simulink model "Modelo_Fuzzy_Manual"  (R2015b)
settings: Solver=ode1  StartTime=0.0  StopTime=tfin  FixedStep=0.05  RelTol=1e-5  AbsTol=1e-15
undefined symbols (not defined in the file): ACSP, ILSnoise, ParamFuzzy, wind
(part 1 of 2)
settings Model: Creator=cpoh  LastModifiedBy=CPOH

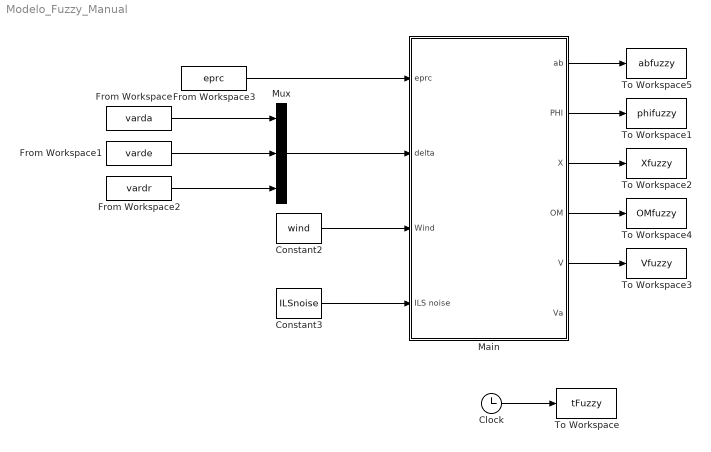
== system Modelo_Fuzzy_Manual ==
  Clock : Clock
  Constant2 : Constant  Value=wind
  Constant3 : Constant  Value=ILSnoise
  From Workspace : FromWorkspace  VariableName=varda  SampleTime=0.05
  From Workspace1 : FromWorkspace  VariableName=varde  SampleTime=0.05
  From Workspace2 : FromWorkspace  VariableName=vardr  SampleTime=0.05
  From Workspace3 : FromWorkspace  VariableName=eprc  SampleTime=0.05
  Main : Subsystem
  Mux : Mux  Inputs=3
  To Workspace : ToWorkspace  VariableName=tFuzzy  SampleTime=-1
  To Workspace1 : ToWorkspace  VariableName=phifuzzy  SampleTime=-1
  To Workspace2 : ToWorkspace  VariableName=Xfuzzy  SampleTime=-1
  To Workspace3 : ToWorkspace  VariableName=Vfuzzy  SampleTime=-1
  To Workspace4 : ToWorkspace  VariableName=OMfuzzy  SampleTime=-1
  To Workspace5 : ToWorkspace  VariableName=abfuzzy  SampleTime=-1
  wires:
  Clock/1 -> To Workspace/1
  Main/2(PHI) -> To Workspace1/1
  Constant3/1 -> Main/4(ILS noise)
  Constant2/1 -> Main/3(Wind)
  Mux/1 -> Main/2(delta)
  From Workspace2/1 -> Mux/3
  From Workspace1/1 -> Mux/2
  From Workspace/1 -> Mux/1
  From Workspace3/1 -> Main/1(eprc)
  Main/3(X) -> To Workspace2/1
  Main/5(V) -> To Workspace3/1
  Main/4(OM) -> To Workspace4/1
  Main/1(ab) -> To Workspace5/1

== system Modelo_Fuzzy_Manual/Main ==
  eprc : Inport
  delta : Inport  Port=2
  Wind : Inport  Port=3
  ILS noise : Inport  Port=4
  A310 Model : Subsystem
  Engines and Actuators : Subsystem
  Gb : Constant  Value=ACSP.U0.wind
  Sum3 : Sum  Inputs=++|
  ab : Outport
  PHI : Outport  Port=2
  X : Outport  Port=3
  OM : Outport  Port=4
  V : Outport  Port=5
  Va : Outport  Port=6
  wires:
  eprc/1 -> Engines and Actuators/1(eprc)
  delta/1 -> Engines and Actuators/2(deflections)
  Engines and Actuators/1(states) -> [xEA]
  Engines and Actuators/2(U) -> A310 Model/1(U)
  Wind/1 -> Sum3/2
  Sum3/1 -> A310 Model/2(Wind)
  Gb/1 -> Sum3/1
  ILS noise/1 -> A310 Model/3(ILSnoise)
  A310 Model/3(PHI) -> PHI/1
  A310 Model/7(Va) -> Va/1
  A310 Model/6(V) -> V/1
  A310 Model/5(OM) -> OM/1
  A310 Model/4(X) -> X/1
  A310 Model/1(ab) -> ab/1

== system Modelo_Fuzzy_Manual/Main/A310 Model ==
  U : Inport
  Wind : Inport  Port=2
  ILSnoise : Inport  Port=3
  Dynamics : Subsystem
  Forces and Momments : Subsystem
  Kinematics : Subsystem
  Mux : Mux  Inputs=2
  Selector10 : Selector  InputPortWidth=3  IndexOptions=Index vector (dialog)  Indices=3  OutputSizes=1
  Trajectory : Subsystem
  WIND : Subsystem
  quat 2 PHI : Subsystem
  ab : Outport
  Nxyz : Outport  Port=2
  PHI : Outport  Port=3
  X : Outport  Port=4
  OM : Outport  Port=5
  V : Outport  Port=6
  Va : Outport  Port=7
  wires:
  Forces and Momments/1(F) -> Dynamics/1(F)
  Forces and Momments/3(M) -> Dynamics/2(M)
  Dynamics/1(V) -> V/1, WIND/1(V), Kinematics/1(V)
  Dynamics/2(OM) -> OM/1, Trajectory/5(OM), Forces and Momments/6(OM), Kinematics/2(OM)
  WIND/1(alpha) -> Mux/1
  WIND/2(beta) -> Mux/2
  Mux/1 -> ab/1, Forces and Momments/1(ab)
  U/1 -> Forces and Momments/2(U)
  WIND/3(Va) -> Va/1, Forces and Momments/3(Va)
  Wind/1 -> WIND/2(WIND)
  WIND/4(qd) -> Forces and Momments/4(qd)
  Kinematics/2(Xdot) -> Trajectory/3(Xdot)
  Kinematics/1(X) -> X/1, Trajectory/2(X)
  Kinematics/3(Quat) -> quat 2 PHI/1(quat)
  ILSnoise/1 -> Trajectory/1(ILSnoise)
  quat 2 PHI/1(PHI) -> PHI/1, Trajectory/4(PHI)
  Forces and Momments/2(Nxyz) -> Nxyz/1
  Selector10/1 -> Forces and Momments/5(HLG)
  Trajectory/2(xyzLG) -> Selector10/1

== system Modelo_Fuzzy_Manual/Main/Engines and Actuators ==
  eprc : Inport
  deflections : Inport  Port=2
  Actuators : Subsystem
  Engines : Subsystem
  Mux : Mux  Inputs=2
  Mux1 : Mux  Inputs=2
  Scope : Scope  NumInputPorts=2
  Sum3 : Sum  Inputs=|++
  delta0 : Constant  Value=ACSP.U0.delta
  epr0 : Constant  Value=ACSP.U0.epr
  states : Outport
  U : Outport  Port=2
  wires:
  Actuators/1(delta) -> Sum3/1, Mux1/2
  Engines/1(TH) -> Mux/1
  eprc/1 -> Engines/2(eprc)
  deflections/1 -> Actuators/1(deltac)
  epr0/1 -> Engines/1(epr0)
  Mux/1 -> U/1
  Engines/2(epr) -> Mux1/1  "EPR"
  Mux1/1 -> states/1
  Sum3/1 -> Scope/1, Mux/2
  delta0/1 -> Sum3/2

== system Modelo_Fuzzy_Manual/Main/A310 Model/Dynamics ==
  note: F =mass*(Vdot + OM x V)
  note: M = I*OMdot + OM x (I*OM)
  F : Inport
  M : Inport  Port=2
  CP1 : Subsystem
      mask Display:
      | fprintf('CROSS \n PRODUCT');
      | color('red');
      | fprintf('\n\n');
      | fprintf(' \n \n \n z=x^y');
      | %text(3,1,'PRODUCT');
      | %text(5,1,'z=x^y');
  CP2 : Subsystem
      mask Display:
      | fprintf('CROSS \n PRODUCT');
      | color('red');
      | fprintf('\n\n');
      | fprintf(' \n \n \n z=x^y');
      | %text(3,1,'PRODUCT');
      | %text(5,1,'z=x^y');
  Inertia : Gain  Gain=ACSP.MIG.I  Multiplication=Matrix(K*u)
  Inertia^-1 : Gain  Gain=ACSP.MIG.J  Multiplication=Matrix(K*u)
  Int_OM : Integrator  InitialCondition=ACSP.X0.OM  ContinuousStateAttributes='OM'
  Int_V : Integrator  InitialCondition=ACSP.X0.V  ContinuousStateAttributes='V'
  Mass^-1 : Gain  Gain=1/ACSP.MIG.mass
  Sum : Sum  Inputs=|+-
  Sum1 : Sum  Inputs=-+|
  V : Outport
  OM : Outport  Port=2
  wires:
  Int_V/1 -> CP2/2(y), V/1
  Sum1/1 -> Int_V/1
  Sum/1 -> Inertia^-1/1
  M/1 -> Sum/1
  Inertia^-1/1 -> Int_OM/1
  F/1 -> Mass^-1/1
  Int_OM/1 -> CP1/1(x), Inertia/1, CP2/1(x), OM/1
  CP2/1(z) -> Sum1/1
  CP1/1(z) -> Sum/2
  Mass^-1/1 -> Sum1/2
  Inertia/1 -> CP1/2(y)

== system Modelo_Fuzzy_Manual/Main/A310 Model/Forces and Momments ==
  ab : Inport
  U : Inport  Port=2
  Va : Inport  Port=3
  qd : Inport  Port=4
  HLG : Inport  Port=5
  OM : Inport  Port=6
  Bus Creator : BusCreator  Inputs=10
  Demux1 : Demux  Outputs=3
  Demux2 : Demux  Outputs=3
  Demux3 : Demux  Outputs=2
  Forces : Subsystem
  Moments : Subsystem
  S : Gain  Gain=ACSP.MIG.Sref
  Selector : Selector  InputPortWidth=4  IndexOptions=Index vector (dialog)  Indices=[2 3 4]  OutputSizes=1
  Selector1 : Selector  InputPortWidth=4  IndexOptions=Index vector (dialog)  Indices=[1]  OutputSizes=1
  F : Outport
  Nxyz : Outport  Port=2
  M : Outport  Port=3
  wires:
  Forces/3(Nxyz) -> Nxyz/1
  Selector1/1 -> Moments/4(TH), Forces/2(TH)
  Forces/2(F) -> F/1
  S/1 -> Moments/3(qS), Forces/3(qS)
  Forces/1(Fa) -> Moments/2(Fa)
  U/1 -> Selector/1, Selector1/1
  Selector/1 -> Demux2/1
  Moments/1(M) -> M/1
  Bus Creator/1 -> Moments/1(E), Forces/1(E)
  Demux1/1 -> Bus Creator/3  "p"
  Demux1/2 -> Bus Creator/4  "q"
  Demux1/3 -> Bus Creator/5  "r"
  Demux3/2 -> Bus Creator/2  "beta"
  Demux2/3 -> Bus Creator/10  "dr"
  Demux2/2 -> Bus Creator/9  "de"
  Demux2/1 -> Bus Creator/8  "da"
  Va/1 -> Bus Creator/6  "Va"
  HLG/1 -> Bus Creator/7  "Hlg"
  OM/1 -> Demux1/1
  qd/1 -> S/1
  Demux3/1 -> Bus Creator/1  "alpha"
  ab/1 -> Demux3/1  "alpha"

== system Modelo_Fuzzy_Manual/Main/A310 Model/Kinematics ==
  V : Inport
  OM : Inport  Port=2
  Gain : Gain  Gain=0.5
  Int_PHI1 : Integrator  InitialCondition=ACSP.X0.QUAT  ContinuousStateAttributes='QUAT'
  Int_X1 : Integrator  InitialCondition=ACSP.X0.X  ContinuousStateAttributes='X'
  R(QUAT) : Subsystem
      mask Display:
      | fprintf('MATRIX \n PRODUCT');
      | color('red');
      | fprintf('\n\n');
      | fprintf(' \n \n \n z=M(x)*y');
  Rotations and transformations matrices in quaternions : Subsystem
  T(QUAT) : Subsystem
      mask Display:
      | fprintf('MATRIX \n PRODUCT');
      | color('red');
      | fprintf('\n\n');
      | fprintf(' \n \n \n z=M(x)*y');
  X : Outport
  Xdot : Outport  Port=2
  Quat : Outport  Port=3
  tag scope: QV2B=global
  wires:
  Int_PHI1/1 -> Quat/1, Rotations and transformations matrices in quaternions/1(QUAT)
  R(QUAT)/1(z) -> Xdot/1, Int_X1/1
  Rotations and transformations matrices in quaternions/3(QB2V) -> R(QUAT)/1(x)
  Rotations and transformations matrices in quaternions/1(TQUAT) -> T(QUAT)/1(x)
  Rotations and transformations matrices in quaternions/2(QV2B) -> [QV2B]
  Gain/1 -> Int_PHI1/1
  T(QUAT)/1(z) -> Gain/1
  OM/1 -> T(QUAT)/2(y)
  V/1 -> R(QUAT)/2(y)
  Int_X1/1 -> X/1

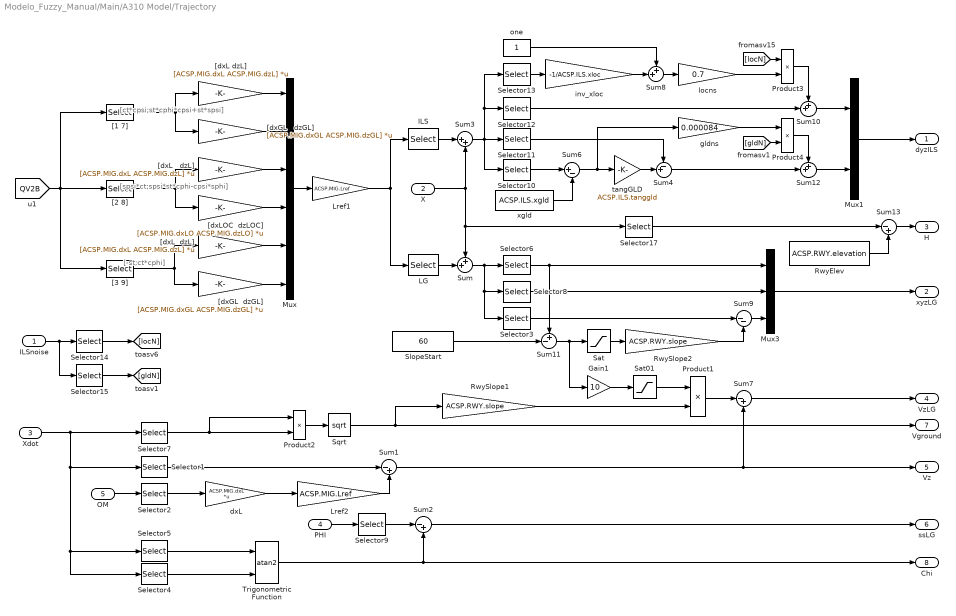
== system Modelo_Fuzzy_Manual/Main/A310 Model/Trajectory ==
  note: [-st;ct*cphi]
  note: [ct*cpsi;st*cphi*cpsi+st*spsi]
  note: [spsi*ct;spsi*st*cphi-cpsi*sphi]
  ILSnoise : Inport
  X : Inport  Port=2
  Xdot : Inport  Port=3
  PHI : Inport  Port=4
  OM : Inport  Port=5
  Gain1 : Gain  Gain=10
  ILS : Selector  InputPortWidth=6  IndexOptions=Index vector (dialog)  Indices=[2 4 6]  OutputSizes=1
  LG : Selector  InputPortWidth=6  IndexOptions=Index vector (dialog)  Indices=[1 3 5]  OutputSizes=1
  Lref1 : Gain  Gain=ACSP.MIG.Lref
  Lref2 : Gain  Gain=ACSP.MIG.Lref
  Mux : Mux  Inputs=6
  Mux1 : Mux  Inputs=2
  Mux3 : Mux  Inputs=3
  Product{1..4} (4 alike) : Product  SaturateOnIntegerOverflow=on  RndMeth=Zero  InputSameDT=on  OutDataTypeStr=Inherit: Same as first input
  RwyElev : Constant  Value=ACSP.RWY.elevation
  RwySlope1 : Gain  Gain=ACSP.RWY.slope
  RwySlope2 : Gain  Gain=ACSP.RWY.slope
  Sat : Saturate  UpperLimit=1000  LowerLimit=0
  Sat01 : Saturate  UpperLimit=1  LowerLimit=0
  Selector{1,3,9,11,17} (5 alike) : Selector  InputPortWidth=3  IndexOptions=Index vector (dialog)  Indices=3  OutputSizes=1
  Selector{4,6..7,10,13} (5 alike) : Selector  InputPortWidth=3  IndexOptions=Index vector (dialog)  Indices=1  OutputSizes=1
  Selector{2,5,8,12} (4 alike) : Selector  InputPortWidth=3  IndexOptions=Index vector (dialog)  Indices=2  OutputSizes=1
  Selector14 : Selector  InputPortWidth=2  IndexOptions=Index vector (dialog)  Indices=1  OutputSizes=1
  Selector15 : Selector  InputPortWidth=2  IndexOptions=Index vector (dialog)  Indices=2  OutputSizes=1
  SlopeStart : Constant  Value=60
  Sqrt : Sqrt  SaturateOnIntegerOverflow=on
  Sum{,8,10,12} (4 alike) : Sum  Inputs=++|
  Sum{1..2,7,13} (4 alike) : Sum  Inputs=|-+
  Sum11 : Sum  Inputs=+-|
  Sum3 : Sum  Inputs=|++
  Sum4 : Sum  Inputs=-+|
  Sum6 : Sum  Inputs=|+-
  Sum9 : Sum  Inputs=|--
  Trigonometric Function : Trigonometry  Operator=atan2
  "[1 7]" : Selector  InputPortWidth=9  IndexOptions=Index vector (dialog)  Indices=[1 7]  OutputSizes=1
  "[2 8]" : Selector  InputPortWidth=9  IndexOptions=Index vector (dialog)  Indices=[2 8]  OutputSizes=1
  "[3 9]" : Selector  InputPortWidth=9  IndexOptions=Index vector (dialog)  Indices=[3 9]  OutputSizes=1
  "[dxGL   dzGL]" : Gain  Gain=[ACSP.MIG.dxGL ACSP.MIG.dzGL]  Multiplication=Matrix(K*u)
  "[dxGL  dzGL]" : Gain  Gain=[ACSP.MIG.dxGL ACSP.MIG.dzGL]  Multiplication=Matrix(K*u)
  "[dxL   dzL]" : Gain  Gain=[ACSP.MIG.dxL ACSP.MIG.dzL]  Multiplication=Matrix(K*u)
  "[dxL  dzL]" : Gain  Gain=[ACSP.MIG.dxL ACSP.MIG.dzL]  Multiplication=Matrix(K*u)
  "[dxL dzL]" : Gain  Gain=[ACSP.MIG.dxL ACSP.MIG.dzL]  Multiplication=Matrix(K*u)
  "[dxLOC  dzLOC]" : Gain  Gain=[ACSP.MIG.dxLO ACSP.MIG.dzLO]  Multiplication=Matrix(K*u)
  dxL : Gain  Gain=ACSP.MIG.dxL  Multiplication=Matrix(K*u)
  gldns : Gain  Gain=0.000084
  inv_xloc : Gain  Gain=-1/ACSP.ILS.xloc
  locns : Gain  Gain=0.7
  one : Constant
  tangGLD : Gain  Gain=ACSP.ILS.tanggld
  xgld : Constant  Value=ACSP.ILS.xgld
  dyzILS : Outport
  xyzLG : Outport  Port=2
  H : Outport  Port=3
  VzLG : Outport  Port=4
  Vz : Outport  Port=5
  ssLG : Outport  Port=6
  Vground : Outport  Port=7
  Chi : Outport  Port=8
  wires:
  Xdot/1 -> Selector1/1, Selector4/1, Selector5/1, Selector7/1
  OM/1 -> Selector2/1
  Selector2/1 -> dxL/1
  dxL/1 -> Lref2/1
  Lref2/1 -> Sum1/2
  Sum1/1 -> Vz/1, Sum7/2
  [QV2B] -> "[1 7]"/1, "[3 9]"/1, "[2 8]"/1
  Selector1/1 -> Sum1/1
  Selector5/1 -> Trigonometric Function/1
  Trigonometric Function/1 -> Sum2/2, Chi/1
  "[1 7]"/1 -> "[dxL dzL]"/1, "[dxGL   dzGL]"/1
  Product2/1 -> Sqrt/1
  Selector4/1 -> Trigonometric Function/2
  Selector7/1 -> Product2/2, Product2/1
  Sqrt/1 -> Vground/1, RwySlope1/1
  "[2 8]"/1 -> "[dxL   dzL]"/1, "[dxLOC  dzLOC]"/1
  PHI/1 -> Selector9/1
  Selector9/1 -> Sum2/1
  Sum2/1 -> ssLG/1
  "[3 9]"/1 -> "[dxL  dzL]"/1, "[dxGL  dzGL]"/1
  "[dxL dzL]"/1 -> Mux/1
  "[dxGL   dzGL]"/1 -> Mux/2
  "[dxL   dzL]"/1 -> Mux/3
  "[dxLOC  dzLOC]"/1 -> Mux/4
  "[dxL  dzL]"/1 -> Mux/5
  "[dxGL  dzGL]"/1 -> Mux/6
  Mux/1 -> Lref1/1
  Lref1/1 -> LG/1, ILS/1
  ILS/1 -> Sum3/1
  Sum3/1 -> Selector10/1, Selector11/1, Selector12/1, Selector13/1
  Sum6/1 -> gldns/1, tangGLD/1
  Selector10/1 -> Sum6/1
  xgld/1 -> Sum6/2
  Mux1/1 -> dyzILS/1
  Selector12/1 -> Sum10/2
  Selector11/1 -> Sum4/1
  tangGLD/1 -> Sum4/2
  Sum4/1 -> Sum12/2
  LG/1 -> Sum/2
  X/1 -> Selector17/1, Sum/1, Sum3/2
  Sum/1 -> Selector6/1, Selector3/1, Selector8/1
  Sat01/1 -> Product1/1
  RwySlope1/1 -> Product1/2
  Sum11/1 -> Gain1/1, Sat/1
  Product1/1 -> Sum7/1
  Sat/1 -> RwySlope2/1
  Mux3/1 -> xyzLG/1
  Selector8/1 -> Mux3/2
  Selector6/1 -> Sum11/1, Mux3/1
  SlopeStart/1 -> Sum11/2
  Sum7/1 -> VzLG/1
  Gain1/1 -> Sat01/1
  Selector13/1 -> inv_xloc/1
  inv_xloc/1 -> Sum8/2
  one/1 -> Sum8/1
  Sum8/1 -> locns/1
  Sum10/1 -> Mux1/1
  locns/1 -> Product3/2
  Product3/1 -> Sum10/1
  Sum12/1 -> Mux1/2
  Product4/1 -> Sum12/1
  gldns/1 -> Product4/1
  ILSnoise/1 -> Selector15/1, Selector14/1
  Selector14/1 -> [locN]
  Selector15/1 -> [gldN]
  [locN] -> Product3/1
  [gldN] -> Product4/2
  RwyElev/1 -> Sum13/2
  Sum13/1 -> H/1
  Selector17/1 -> Sum13/1
  Sum9/1 -> Mux3/3
  RwySlope2/1 -> Sum9/2
  Selector3/1 -> Sum9/1

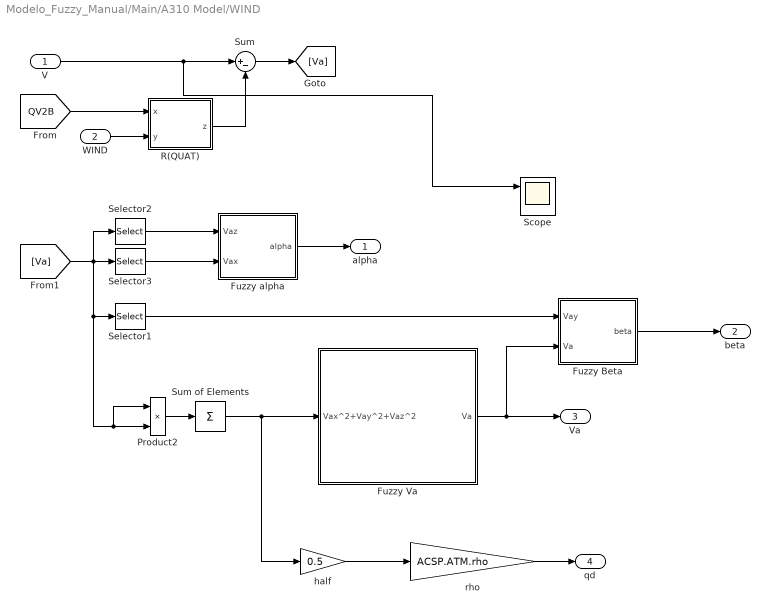
== system Modelo_Fuzzy_Manual/Main/A310 Model/WIND ==
  V : Inport
  WIND : Inport  Port=2
  Fuzzy Beta : Subsystem
  Fuzzy Va : Subsystem
  Fuzzy alpha : Subsystem
  Product2 : Product  SaturateOnIntegerOverflow=on  RndMeth=Zero  InputSameDT=on  OutDataTypeStr=Inherit: Same as first input
  R(QUAT) : Subsystem
      mask Display:
      | fprintf('MATRIX \n PRODUCT');
      | color('red');
      | fprintf('\n\n');
      | fprintf(' \n \n \n z=M(x)*y');
  Scope : Scope  NumInputPorts=2
  Selector1 : Selector  InputPortWidth=3  IndexOptions=Index vector (dialog)  Indices=2  OutputSizes=1
  Selector2 : Selector  InputPortWidth=3  IndexOptions=Index vector (dialog)  Indices=3  OutputSizes=1
  Selector3 : Selector  InputPortWidth=3  IndexOptions=Index vector (dialog)  Indices=1  OutputSizes=1
  Sum : Sum  Inputs=|+-
  Sum of Elements : Sum  Inputs=+
  half : Gain  Gain=0.5  SaturateOnIntegerOverflow=on  OutDataTypeStr=Inherit: Same as input  ParamDataTypeStr=Inherit: Same as input
  rho : Gain  Gain=ACSP.ATM.rho
  alpha : Outport
  beta : Outport  Port=2
  Va : Outport  Port=3
  qd : Outport  Port=4
  wires:
  [QV2B] -> R(QUAT)/1(x)
  WIND/1 -> R(QUAT)/2(y)
  V/1 -> Scope/1, Sum/1
  R(QUAT)/1(z) -> Sum/2
  Sum/1 -> [Va]
  [Va] -> Product2/1, Product2/2, Selector1/1, Selector3/1, Selector2/1
  Product2/1 -> Sum of Elements/1
  Sum of Elements/1 -> half/1, Fuzzy Va/1(Vax^2+Vay^2+Vaz^2)
  Fuzzy Va/1(Va) -> Fuzzy Beta/2(Va), Va/1
  rho/1 -> qd/1
  half/1 -> rho/1
  Selector1/1 -> Fuzzy Beta/1(Vay)
  Fuzzy Beta/1(beta) -> beta/1
  Selector2/1 -> Fuzzy alpha/1(Vaz)
  Selector3/1 -> Fuzzy alpha/2(Vax)
  Fuzzy alpha/1(alpha) -> alpha/1

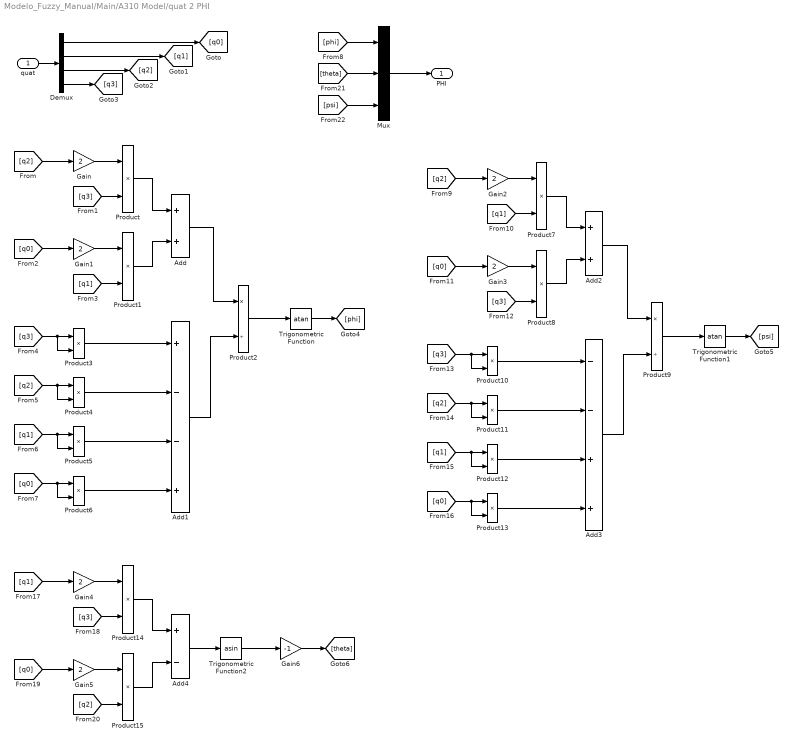
== system Modelo_Fuzzy_Manual/Main/A310 Model/quat 2 PHI ==
  quat : Inport
  Add : Sum
  Add1 : Sum  Inputs=+--+
  Add2 : Sum
  Add3 : Sum  Inputs=--++
  Add4 : Sum  Inputs=+-
  Demux : Demux
  Gain{,1..5} (6 alike) : Gain  Gain=2
  Gain6 : Gain  Gain=-1
  Mux : Mux  Inputs=3
  Product{,1,3..8,10..15} (14 alike) : Product
  Product2 : Product  Inputs=*/
  Product9 : Product  Inputs=*/
  Trigonometric Function : Trigonometry  Operator=atan
  Trigonometric Function1 : Trigonometry  Operator=atan
  Trigonometric Function2 : Trigonometry  Operator=asin
  PHI : Outport
  wires:
  quat/1 -> Demux/1
  Demux/1 -> [q0]
  Demux/2 -> [q1]
  Demux/3 -> [q2]
  Demux/4 -> [q3]
  [q3] -> Product/2
  Gain/1 -> Product/1
  [q2] -> Gain/1
  [q1] -> Product1/2
  Gain1/1 -> Product1/1
  [q0] -> Gain1/1
  Product/1 -> Add/1
  Product1/1 -> Add/2
  [q3] -> Product3/2, Product3/1
  [q2] -> Product4/2, Product4/1
  [q1] -> Product5/2, Product5/1
  [q0] -> Product6/2, Product6/1
  Product3/1 -> Add1/1
  Product4/1 -> Add1/2
  Product5/1 -> Add1/3
  Product6/1 -> Add1/4
  Add1/1 -> Product2/2
  Add/1 -> Product2/1
  Product2/1 -> Trigonometric Function/1
  Trigonometric Function/1 -> [phi]
  Mux/1 -> PHI/1
  [phi] -> Mux/1
  [q1] -> Product7/2
  Gain2/1 -> Product7/1
  [q2] -> Gain2/1
  [q3] -> Product8/2
  Gain3/1 -> Product8/1
  [q0] -> Gain3/1
  Product7/1 -> Add2/1
  Product8/1 -> Add2/2
  [q3] -> Product10/2, Product10/1
  [q2] -> Product11/2, Product11/1
  [q1] -> Product12/2, Product12/1
  [q0] -> Product13/2, Product13/1
  Product10/1 -> Add3/1
  Product11/1 -> Add3/2
  Product12/1 -> Add3/3
  Product13/1 -> Add3/4
  Add3/1 -> Product9/2
  Add2/1 -> Product9/1
  Product9/1 -> Trigonometric Function1/1
  Trigonometric Function1/1 -> [psi]
  [q3] -> Product14/2
  Gain4/1 -> Product14/1
  [q1] -> Gain4/1
  [q2] -> Product15/2
  Gain5/1 -> Product15/1
  [q0] -> Gain5/1
  Product14/1 -> Add4/1
  Product15/1 -> Add4/2
  Add4/1 -> Trigonometric Function2/1
  Trigonometric Function2/1 -> Gain6/1
  Gain6/1 -> [theta]
  [theta] -> Mux/2
  [psi] -> Mux/3

== system Modelo_Fuzzy_Manual/Main/Engines and Actuators/Actuators ==
  deltac : Inport
  Gain2 : Gain  Gain=1./ACSP.ACT.tau
  Int_ASD : Integrator  ContinuousStateAttributes='xASD'
  ML [55 25 30] : Saturate  UpperLimit=ACSP.ACT.ML  LowerLimit=-ACSP.ACT.ML
  RL [60 20 30] : Saturate  UpperLimit=ACSP.ACT.RL  LowerLimit=-ACSP.ACT.RL
  Sum : Sum  Inputs=|+-
  delta : Outport
  wires:
  ML [55 25 30]/1 -> delta/1
  Sum/1 -> Gain2/1
  deltac/1 -> Sum/1
  Int_ASD/1 -> ML [55 25 30]/1, Sum/2
  RL [60 20 30]/1 -> Int_ASD/1
  Gain2/1 -> RL [60 20 30]/1

== system Modelo_Fuzzy_Manual/Main/Engines and Actuators/Engines ==
  epr0 : Inport
  eprc : Inport  Port=2
  EML : Saturate  UpperLimit=ACSP.ENG.UML  LowerLimit=ACSP.ENG.LML
  ERL : Saturate  UpperLimit=ACSP.ENG.RL  LowerLimit=-ACSP.ENG.RL
  Gain1 : Gain  Gain=1/ACSP.ENG.tau
  Gain2 : Gain  Gain=ACSP.ENG.Ga
  Gb : Constant  Value=ACSP.ENG.Gb
  Int_ENG : Integrator  ContinuousStateAttributes='xENG'
  Sum : Sum  Inputs=|+-
  Sum1 : Sum  Inputs=+-|
  Sum2 : Sum  Inputs=|++
  Sum3 : Sum  Inputs=++|
  TH : Outport
  epr : Outport  Port=2
  wires:
  Sum2/1 -> EML/1
  Gb/1 -> Sum3/1
  Gain2/1 -> Sum3/2
  Sum3/1 -> TH/1
  eprc/1 -> Sum/1
  Int_ENG/1 -> Sum2/1, Sum/2
  ERL/1 -> Int_ENG/1
  Gain1/1 -> ERL/1
  Sum/1 -> Gain1/1
  EML/1 -> Sum1/1, Gain2/1
  epr0/1 -> Sum1/2, Sum2/2
  Sum1/1 -> epr/1

== system Modelo_Fuzzy_Manual/Main/A310 Model/Dynamics/CP1 ==
  x : Inport
  y : Inport  Port=2
  Mux : Mux  Inputs=2
  Mux1 : Mux  Inputs=3
  Y1 : Fcn  Expr=u(2)*u(6)-u(3)*u(5)
  Y2 : Fcn  Expr=u(3)*u(4)-u(1)*u(6)
  Y3 : Fcn  Expr=u(1)*u(5)-u(2)*u(4)
  z : Outport
  wires:
  Mux1/1 -> z/1
  Y2/1 -> Mux1/2
  Y1/1 -> Mux1/1
  Y3/1 -> Mux1/3
  y/1 -> Mux/2
  Mux/1 -> Y2/1, Y3/1, Y1/1
  x/1 -> Mux/1

== system Modelo_Fuzzy_Manual/Main/A310 Model/Dynamics/CP2 ==
  x : Inport
  y : Inport  Port=2
  Mux : Mux  Inputs=2
  Mux1 : Mux  Inputs=3
  Y1 : Fcn  Expr=u(2)*u(6)-u(3)*u(5)
  Y2 : Fcn  Expr=u(3)*u(4)-u(1)*u(6)
  Y3 : Fcn  Expr=u(1)*u(5)-u(2)*u(4)
  z : Outport
  wires:
  Mux1/1 -> z/1
  Y2/1 -> Mux1/2
  Y1/1 -> Mux1/1
  Y3/1 -> Mux1/3
  y/1 -> Mux/2
  Mux/1 -> Y2/1, Y3/1, Y1/1
  x/1 -> Mux/1

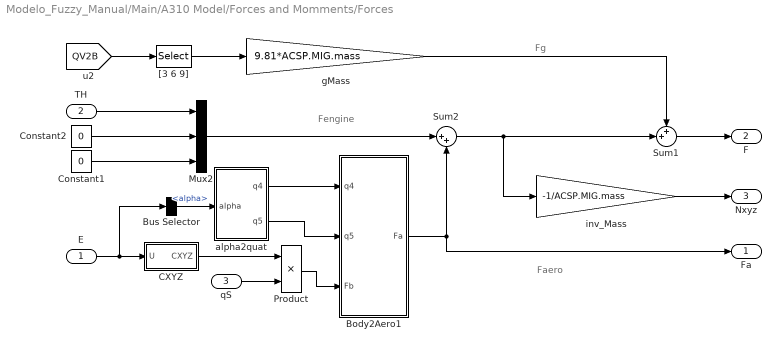
== system Modelo_Fuzzy_Manual/Main/A310 Model/Forces and Momments/Forces ==
  note: Fg
  note: Fengine
  note: Faero
  E : Inport
  TH : Inport  Port=2
  qS : Inport  Port=3
  Body2Aero1 : Subsystem
  Bus Selector : BusSelector  OutputSignals=alpha
  CXYZ : Subsystem
  Constant1 : Constant  Value=0
  Constant2 : Constant  Value=0
  Mux2 : Mux  Inputs=3
  Product : Product  RndMeth=Zero
  Sum1 : Sum  Inputs=++|
  Sum2 : Sum  Inputs=|++
  "[3 6 9]" : Selector  InputPortWidth=9  IndexOptions=Index vector (dialog)  Indices=[3 6 9]  OutputSizes=1
  alpha2quat : Subsystem
  gMass : Gain  Gain=9.81*ACSP.MIG.mass
  inv_Mass : Gain  Gain=-1/ACSP.MIG.mass
  Fa : Outport
  F : Outport  Port=2
  Nxyz : Outport  Port=3
  wires:
  inv_Mass/1 -> Nxyz/1
  Sum2/1 -> Sum1/2, inv_Mass/1
  Mux2/1 -> Sum2/1
  CXYZ/1(CXYZ) -> Product/1
  E/1 -> CXYZ/1(U), Bus Selector/1
  Product/1 -> Body2Aero1/3(Fb)
  qS/1 -> Product/2
  Sum1/1 -> F/1
  "[3 6 9]"/1 -> gMass/1
  [QV2B] -> "[3 6 9]"/1
  Constant1/1 -> Mux2/3
  Constant2/1 -> Mux2/2
  TH/1 -> Mux2/1
  Bus Selector/1 -> alpha2quat/1(alpha)  "<alpha>"
  alpha2quat/1(q4) -> Body2Aero1/1(q4)
  alpha2quat/2(q5) -> Body2Aero1/2(q5)
  gMass/1 -> Sum1/1
  Body2Aero1/1(Fa) -> Fa/1, Sum2/2

== system Modelo_Fuzzy_Manual/Main/A310 Model/Forces and Momments/Moments ==
  note: Ma
  note: Mengine
  note: MFaero
  E : Inport
  Fa : Inport  Port=2
  qS : Inport  Port=3
  TH : Inport  Port=4
  CD0 : Constant  Value=ACSP.MIG.dxG
  CP : Subsystem
      mask Display:
      | fprintf('CROSS \n PRODUCT');
      | color('red');
      | fprintf('\n\n');
      | fprintf(' \n \n \n z=x^y');
      | %text(3,1,'PRODUCT');
      | %text(5,1,'z=x^y');
  Clmn : Subsystem
  Constant{1..4} (4 alike) : Constant  Value=0
  Engine vertical position : Gain  Gain=ACSP.MIG.dzE
  Lref : Gain  Gain=ACSP.MIG.Lref
  Mux1 : Mux  Inputs=3
  Mux2 : Mux  Inputs=3
  Product : Product  RndMeth=Zero
  Sum1 : Sum  Inputs=+++
  M : Outport
  wires:
  E/1 -> Clmn/1(U)
  Clmn/1(Clmn) -> Product/2
  Lref/1 -> M/1
  Mux2/1 -> Sum1/3
  Product/1 -> Sum1/2
  CD0/1 -> Mux1/1
  Constant4/1 -> Mux1/3
  Constant3/1 -> Mux1/2
  CP/1(z) -> Sum1/1
  Mux1/1 -> CP/1(x)
  Fa/1 -> CP/2(y)
  qS/1 -> Product/1
  Constant2/1 -> Mux2/1
  Engine vertical position/1 -> Mux2/2
  TH/1 -> Engine vertical position/1
  Sum1/1 -> Lref/1
  Constant1/1 -> Mux2/3

== system Modelo_Fuzzy_Manual/Main/A310 Model/Kinematics/R(QUAT) ==
  x : Inport
  y : Inport  Port=2
  Mux : Mux  Inputs=2
  Mux1 : Mux  Inputs=3
  Y1 : Fcn  Expr=u(1)*u(10)+u(2)*u(11)+u(3)*u(12)
  Y2 : Fcn  Expr=u(4)*u(10)+u(5)*u(11)+u(6)*u(12)
  Y3 : Fcn  Expr=u(7)*u(10)+u(8)*u(11)+u(9)*u(12)
  z : Outport
  wires:
  Mux1/1 -> z/1
  Y2/1 -> Mux1/2
  Y1/1 -> Mux1/1
  Y3/1 -> Mux1/3
  y/1 -> Mux/2
  Mux/1 -> Y2/1, Y1/1, Y3/1
  x/1 -> Mux/1

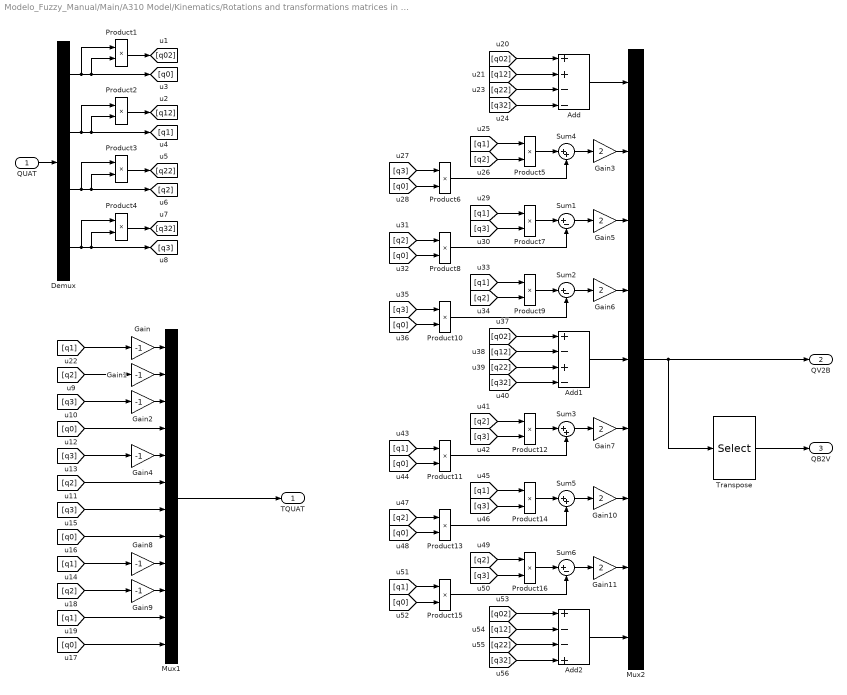
== system Modelo_Fuzzy_Manual/Main/A310 Model/Kinematics/Rotations and transformations matrices in quaternions ==
  QUAT : Inport
  Add : Sum  Inputs=++--
  Add1 : Sum  Inputs=+-+-
  Add2 : Sum  Inputs=+--+
  Demux : Demux
  Gain{,1..2,4,8..9} (6 alike) : Gain  Gain=-1
  Gain{3,5..7,10..11} (6 alike) : Gain  Gain=2
  Mux1 : Mux  Inputs=12
  Mux2 : Mux  Inputs=9
  Product{1..16} (16 alike) : Product  SaturateOnIntegerOverflow=on  RndMeth=Zero  InputSameDT=on  OutDataTypeStr=Inherit: Same as first input
  Sum1 : Sum  Inputs=|+-
  Sum2 : Sum  Inputs=|+-
  Sum3 : Sum  Inputs=|++
  Sum4 : Sum  Inputs=|++
  Sum5 : Sum  Inputs=|++
  Sum6 : Sum  Inputs=|+-
  Transpose : Selector  InputPortWidth=9  IndexOptions=Index vector (dialog)  Indices=[1 4 7 2 5 8 3 6 9]  OutputSizes=1
  TQUAT : Outport
  QV2B : Outport  Port=2
  QB2V : Outport  Port=3
  wires:
  QUAT/1 -> Demux/1
  Demux/1 -> Product1/1, Product1/2, [q0]
  Product1/1 -> [q02]
  Demux/2 -> Product2/1, Product2/2, [q1]
  Product2/1 -> [q12]
  Demux/3 -> Product3/1, Product3/2, [q2]
  Product3/1 -> [q22]
  Demux/4 -> Product4/1, Product4/2, [q3]
  Product4/1 -> [q32]
  Mux1/1 -> TQUAT/1
  Gain/1 -> Mux1/1
  [q1] -> Gain/1
  [q2] -> Gain1/1
  Gain1/1 -> Mux1/2
  [q3] -> Gain2/1
  Gain2/1 -> Mux1/3
  [q3] -> Gain4/1
  [q1] -> Gain8/1
  [q2] -> Gain9/1
  Gain9/1 -> Mux1/10
  [q1] -> Mux1/11
  [q0] -> Mux1/12
  Gain8/1 -> Mux1/9
  [q0] -> Mux1/8
  [q3] -> Mux1/7
  [q2] -> Mux1/6
  Gain4/1 -> Mux1/5
  [q0] -> Mux1/4
  Add/1 -> Mux2/1
  [q32] -> Add/4
  [q22] -> Add/3
  [q12] -> Add/2
  [q02] -> Add/1
  Gain3/1 -> Mux2/2
  Sum4/1 -> Gain3/1
  Product5/1 -> Sum4/1
  [q1] -> Product5/1
  [q2] -> Product5/2
  Product6/1 -> Sum4/2
  [q3] -> Product6/1
  [q0] -> Product6/2
  Gain5/1 -> Mux2/3
  Sum1/1 -> Gain5/1
  Product7/1 -> Sum1/1
  [q1] -> Product7/1
  [q3] -> Product7/2
  Product8/1 -> Sum1/2
  [q2] -> Product8/1
  [q0] -> Product8/2
  Gain6/1 -> Mux2/4
  Sum2/1 -> Gain6/1
  Product9/1 -> Sum2/1
  [q1] -> Product9/1
  [q2] -> Product9/2
  Product10/1 -> Sum2/2
  [q3] -> Product10/1
  [q0] -> Product10/2
  Add1/1 -> Mux2/5
  [q32] -> Add1/4
  [q22] -> Add1/3
  [q12] -> Add1/2
  [q02] -> Add1/1
  Sum3/1 -> Gain7/1
  Product12/1 -> Sum3/1
  [q2] -> Product12/1
  [q3] -> Product12/2
  Product11/1 -> Sum3/2
  [q1] -> Product11/1
  [q0] -> Product11/2
  Gain7/1 -> Mux2/6
  Sum5/1 -> Gain10/1
  Product14/1 -> Sum5/1
  [q1] -> Product14/1
  [q3] -> Product14/2
  Product13/1 -> Sum5/2
  [q2] -> Product13/1
  [q0] -> Product13/2
  Gain10/1 -> Mux2/7
  Sum6/1 -> Gain11/1
  Product16/1 -> Sum6/1
  [q2] -> Product16/1
  [q3] -> Product16/2
  Product15/1 -> Sum6/2
  [q1] -> Product15/1
  [q0] -> Product15/2
  Gain11/1 -> Mux2/8
  Add2/1 -> Mux2/9
  [q32] -> Add2/4
  [q22] -> Add2/3
  [q12] -> Add2/2
  [q02] -> Add2/1
  Mux2/1 -> QV2B/1, Transpose/1
  Transpose/1 -> QB2V/1

== system Modelo_Fuzzy_Manual/Main/A310 Model/Kinematics/T(QUAT) ==
  x : Inport
  y : Inport  Port=2
  Mux : Mux  Inputs=2
  Mux1 : Mux
  Y1 : Fcn  Expr=u(1)*u(13)+u(2)*u(14)+u(3)*u(15)
  Y2 : Fcn  Expr=u(4)*u(13)+u(5)*u(14)+u(6)*u(15)
  Y3 : Fcn  Expr=u(7)*u(13)+u(8)*u(14)+u(9)*u(15)
  Y4 : Fcn  Expr=u(10)*u(13)+u(11)*u(14)+u(12)*u(15)
  z : Outport
  wires:
  Mux1/1 -> z/1
  Y2/1 -> Mux1/2
  Y1/1 -> Mux1/1
  Y3/1 -> Mux1/3
  y/1 -> Mux/2
  Mux/1 -> Y2/1, Y1/1, Y4/1, Y3/1
  x/1 -> Mux/1
  Y4/1 -> Mux1/4

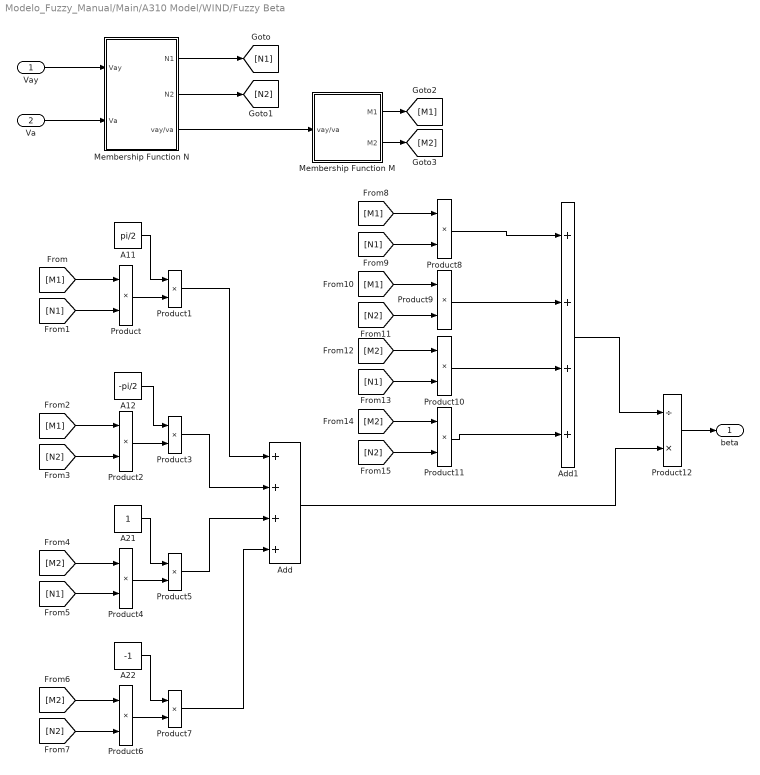
== system Modelo_Fuzzy_Manual/Main/A310 Model/WIND/Fuzzy Beta ==
  Vay : Inport
  Va : Inport  Port=2
  A11 : Constant  Value=pi/2
  A12 : Constant  Value=-pi/2
  A21 : Constant
  A22 : Constant  Value=-1
  Add : Sum  Inputs=++++
  Add1 : Sum  Inputs=++++
  Membership Function M : Subsystem
  Membership Function N : Subsystem
  Product{,1..11} (12 alike) : Product
  Product12 : Product  Inputs=/*
  beta : Outport
  wires:
  Vay/1 -> Membership Function N/1(Vay)
  Va/1 -> Membership Function N/2(Va)
  Membership Function M/2(M2) -> [M2]
  Membership Function M/1(M1) -> [M1]
  Membership Function N/2(N2) -> [N2]
  Membership Function N/1(N1) -> [N1]
  Membership Function N/3(vay/va) -> Membership Function M/1(vay/va)
  A11/1 -> Product1/1
  [M1] -> Product/1
  Product/1 -> Product1/2
  [N1] -> Product/2
  A12/1 -> Product3/1
  [M1] -> Product2/1
  Product2/1 -> Product3/2
  [N2] -> Product2/2
  A21/1 -> Product5/1
  [M2] -> Product4/1
  Product4/1 -> Product5/2
  [N1] -> Product4/2
  A22/1 -> Product7/1
  [M2] -> Product6/1
  Product6/1 -> Product7/2
  [N2] -> Product6/2
  Product1/1 -> Add/1
  Product3/1 -> Add/2
  Product5/1 -> Add/3
  Product7/1 -> Add/4
  [M1] -> Product8/1
  [N1] -> Product8/2
  [M1] -> Product9/1
  [N2] -> Product9/2
  [M2] -> Product11/1
  [N2] -> Product11/2
  Product9/1 -> Add1/2
  Product10/1 -> Add1/3
  Product8/1 -> Add1/1
  Product11/1 -> Add1/4
  Product12/1 -> beta/1
  Add1/1 -> Product12/1
  Add/1 -> Product12/2
  [M2] -> Product10/1
  [N1] -> Product10/2

== system Modelo_Fuzzy_Manual/Main/A310 Model/WIND/Fuzzy Va ==
  Vax^2+Vay^2+Vaz^2 : Inport
  Add : Sum
  Max : Constant  Value=160000
  Membership functions : Subsystem
  Min : Constant  Value=0
  Product : Product
  Product1 : Product
  Va : Outport
  wires:
  Vax^2+Vay^2+Vaz^2/1 -> Membership functions/1(U)
  Max/1 -> Product/1
  Membership functions/1(M1) -> Product/2
  Membership functions/2(M2) -> Product1/1
  Min/1 -> Product1/2
  Product1/1 -> Add/2
  Product/1 -> Add/1
  Add/1 -> Va/1

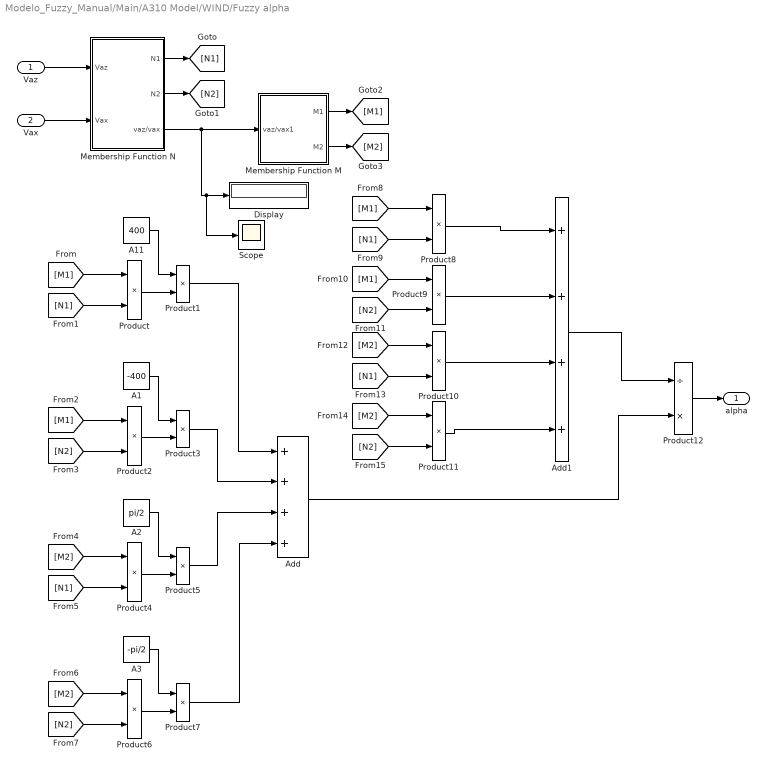
== system Modelo_Fuzzy_Manual/Main/A310 Model/WIND/Fuzzy alpha ==
  Vaz : Inport
  Vax : Inport  Port=2
  A1 : Constant  Value=-400
  A11 : Constant  Value=400
  A2 : Constant  Value=pi/2
  A3 : Constant  Value=-pi/2
  Add : Sum  Inputs=++++
  Add1 : Sum  Inputs=++++
  Display : Display
  Membership Function M : Subsystem
  Membership Function N : Subsystem
  Product{,1..11} (12 alike) : Product
  Product12 : Product  Inputs=/*
  Scope : Scope
  alpha : Outport
  wires:
  Vaz/1 -> Membership Function N/1(Vaz)
  Vax/1 -> Membership Function N/2(Vax)
  Membership Function N/1(N1) -> [N1]
  Membership Function N/2(N2) -> [N2]
  A11/1 -> Product1/1
  [M1] -> Product/1
  Product/1 -> Product1/2
  [N1] -> Product/2
  A1/1 -> Product3/1
  [M1] -> Product2/1
  Product2/1 -> Product3/2
  [N2] -> Product2/2
  A2/1 -> Product5/1
  [M2] -> Product4/1
  Product4/1 -> Product5/2
  [N1] -> Product4/2
  A3/1 -> Product7/1
  [M2] -> Product6/1
  Product6/1 -> Product7/2
  [N2] -> Product6/2
  Product1/1 -> Add/1
  Product3/1 -> Add/2
  Product5/1 -> Add/3
  Product7/1 -> Add/4
  [M1] -> Product8/1
  [N1] -> Product8/2
  [M1] -> Product9/1
  [N2] -> Product9/2
  [M2] -> Product11/1
  Product9/1 -> Add1/2
  Product10/1 -> Add1/3
  Product8/1 -> Add1/1
  Product11/1 -> Add1/4
  Add1/1 -> Product12/1
  Add/1 -> Product12/2
  Product12/1 -> alpha/1
  [N2] -> Product11/2
  [M2] -> Product10/1
  [N1] -> Product10/2
  Membership Function N/3(vaz/vax) -> Scope/1, Display/1, Membership Function M/1(vaz/vax1)
  Membership Function M/1(M1) -> [M1]
  Membership Function M/2(M2) -> [M2]

== system Modelo_Fuzzy_Manual/Main/A310 Model/WIND/R(QUAT) ==
  x : Inport
  y : Inport  Port=2
  Mux : Mux  Inputs=2
  Mux1 : Mux  Inputs=3
  Y1 : Fcn  Expr=u(1)*u(10)+u(2)*u(11)+u(3)*u(12)
  Y2 : Fcn  Expr=u(4)*u(10)+u(5)*u(11)+u(6)*u(12)
  Y3 : Fcn  Expr=u(7)*u(10)+u(8)*u(11)+u(9)*u(12)
  z : Outport
  wires:
  Mux1/1 -> z/1
  Y2/1 -> Mux1/2
  Y1/1 -> Mux1/1
  Y3/1 -> Mux1/3
  y/1 -> Mux/2
  Mux/1 -> Y2/1, Y1/1, Y3/1
  x/1 -> Mux/1

== system Modelo_Fuzzy_Manual/Main/A310 Model/Forces and Momments/Forces/Body2Aero1 ==
  q4 : Inport
  q5 : Inport  Port=2
  Fb : Inport  Port=3
  Mux : Mux  Inputs=[1 1 3]
  Mux3 : Mux  Inputs=3
  Segunda fila : Fcn  Expr=(u(1)^2+u(2)^2)*u(4)
  Tercera fila : Fcn  Expr=-2*u(1)*u(2)*u(3)+(u(1)^2-u(2)^2)*u(5)
  primera fila : Fcn  Expr=(u(1)^2-u(2)^2)*u(3)+2*u(1)*u(2)*u(5)
  Fa : Outport
  wires:
  Fb/1 -> Mux/3
  q4/1 -> Mux/1
  q5/1 -> Mux/2
  Mux/1 -> Tercera fila/1, Segunda fila/1, primera fila/1
  Tercera fila/1 -> Mux3/3
  Segunda fila/1 -> Mux3/2
  primera fila/1 -> Mux3/1
  Mux3/1 -> Fa/1

== system Modelo_Fuzzy_Manual/Main/A310 Model/Forces and Momments/Forces/CXYZ ==
  U : Inport
  Bus Selector : BusSelector  OutputSignals=alpha
  Bus Selector1 : BusSelector  OutputSignals=beta,dr
  Bus Selector2 : BusSelector  OutputSignals=alpha,q,Va,de
  Bus Selector3 : BusSelector  OutputSignals=Hlg
  CL0 : Constant  Value=ACSP.COEF.CL.CL0
  CLa : Gain  Gain=ACSP.COEF.CL.CLa
  CLa3 : Gain  Gain=ACSP.COEF.CL.CLde
  CY_beta : Gain  Gain=ACSP.COEF.CY.CYb
  CY_dr : Gain  Gain=ACSP.COEF.CY.CYdr
  Fuzzy CD (manual) : Subsystem
  Fuzzy CL1 (manual) : Subsystem
  Fuzzy CL2 (manual) : Subsystem
  Gain : Gain  Gain=-1
  Gain1 : Gain  Gain=-1
  Mux : Mux  Inputs=3
  Sum1 : Sum
  Sum3 : Sum  Inputs=++++
  Sum4 : Sum  Inputs=|++
  CXYZ : Outport
  wires:
  Sum4/1 -> Gain1/1
  Sum3/1 -> Sum4/1
  CLa3/1 -> Sum3/4
  Bus Selector2/4 -> CLa3/1  "<de>"
  Mux/1 -> CXYZ/1
  Sum1/1 -> Mux/2
  Gain/1 -> Mux/1
  Gain1/1 -> Mux/3
  CL0/1 -> Sum3/1
  Bus Selector2/1 -> CLa/1  "<alpha>"
  CLa/1 -> Sum3/2
  CY_dr/1 -> Sum1/2
  CY_beta/1 -> Sum1/1
  Bus Selector1/2 -> CY_dr/1  "<dr>"
  Bus Selector1/1 -> CY_beta/1  "<beta>"
  U/1 -> Bus Selector/1, Bus Selector1/1, Bus Selector2/1, Bus Selector3/1
  Bus Selector2/2 -> Fuzzy CL1 (manual)/1(q)  "<q>"
  Bus Selector2/3 -> Fuzzy CL1 (manual)/2(Va)  "<Va>"
  Fuzzy CL1 (manual)/1(CL1) -> Sum3/3
  Bus Selector3/1 -> Fuzzy CL2 (manual)/1(Hlg)  "<Hlg>"
  Fuzzy CL2 (manual)/1(CL2) -> Sum4/2
  Bus Selector/1 -> Fuzzy CD (manual)/1(alpha)  "<alpha>"
  Fuzzy CD (manual)/1(CD) -> Gain/1

== system Modelo_Fuzzy_Manual/Main/A310 Model/Forces and Momments/Forces/alpha2quat ==
  alpha : Inport
  Constant : Constant  Value=-2
  Divide : Product  Inputs=*/
  Trigonometric Function : Trigonometry  Operator=cos
  Trigonometric Function1 : Trigonometry
  q4 : Outport
  q5 : Outport  Port=2
  wires:
  alpha/1 -> Divide/1
  Constant/1 -> Divide/2
  Divide/1 -> Trigonometric Function1/1, Trigonometric Function/1
  Trigonometric Function/1 -> q4/1
  Trigonometric Function1/1 -> q5/1

== system Modelo_Fuzzy_Manual/Main/A310 Model/Forces and Momments/Moments/CP ==
  x : Inport
  y : Inport  Port=2
  Mux : Mux  Inputs=2
  Mux1 : Mux  Inputs=3
  Y1 : Fcn  Expr=u(2)*u(6)-u(3)*u(5)
  Y2 : Fcn  Expr=u(3)*u(4)-u(1)*u(6)
  Y3 : Fcn  Expr=u(1)*u(5)-u(2)*u(4)
  z : Outport
  wires:
  Mux1/1 -> z/1
  Y2/1 -> Mux1/2
  Y1/1 -> Mux1/1
  Y3/1 -> Mux1/3
  y/1 -> Mux/2
  Mux/1 -> Y2/1, Y3/1, Y1/1
  x/1 -> Mux/1

== system Modelo_Fuzzy_Manual/Main/A310 Model/Forces and Momments/Moments/Clmn ==
  U : Inport
  Cl : Subsystem
  Cm : Subsystem
  Cn : Subsystem
  Mux : Mux  Inputs=3
  Clmn : Outport
  wires:
  Mux/1 -> Clmn/1
  Cn/1(Cn) -> Mux/3
  Cm/1(Cm) -> Mux/2
  Cl/1(Cl) -> Mux/1
  U/1 -> Cm/1(U), Cl/1(U), Cn/1(U)

== system Modelo_Fuzzy_Manual/Main/A310 Model/WIND/Fuzzy Beta/Membership Function M ==
  vay/va : Inport
  Add : Sum
  Add1 : Sum
  Constant : Constant
  If : If  IfExpression=u1==0
  If Action Subsystem : Subsystem  TreatAsAtomicUnit=on
  If Action Subsystem1 : Subsystem  TreatAsAtomicUnit=on
  M1 : Outport
  M2 : Outport  Port=2
  wires:
  vay/va/1 -> If Action Subsystem/1(vay/va), If/1
  If/1 -> If Action Subsystem1/Action
  If/2 -> If Action Subsystem/Action
  Constant/1 -> If Action Subsystem1/1(In1)
  If Action Subsystem1/1(M1) -> Add/1
  If Action Subsystem/1(M1) -> Add/2
  If Action Subsystem/2(M2) -> Add1/2
  If Action Subsystem1/2(M2) -> Add1/1
  Add/1 -> M1/1
  Add1/1 -> M2/1

== system Modelo_Fuzzy_Manual/Main/A310 Model/WIND/Fuzzy Beta/Membership Function N ==
  Vay : Inport
  Va : Inport  Port=2
  Add : Sum
  Add1 : Sum  Inputs=-+
  Constant : Constant
  Constant1 : Constant  Value=2
  Constant2 : Constant
  Divide : Product  Inputs=*/
  Divide1 : Product  Inputs=*/
  N1 : Outport
  N2 : Outport  Port=2
  vay/va : Outport  Port=3
  wires:
  Va/1 -> Divide/2
  Vay/1 -> Divide/1
  Divide/1 -> vay/va/1, Add/2
  Constant/1 -> Add/1
  Add/1 -> Divide1/1
  Constant1/1 -> Divide1/2
  Divide1/1 -> Add1/1, N1/1
  Add1/1 -> N2/1
  Constant2/1 -> Add1/2

== system Modelo_Fuzzy_Manual/Main/A310 Model/WIND/Fuzzy Va/Membership functions ==
  U : Inport
  Add : Sum  Inputs=-+
  Constant : Constant  Value=160000
  Constant1 : Constant
  Product : Product  Inputs=*/
  Sqrt : Sqrt  SaturateOnIntegerOverflow=on
  M1 : Outport
  M2 : Outport  Port=2
  wires:
  U/1 -> Sqrt/1
  Sqrt/1 -> Product/1
  Constant/1 -> Product/2
  Product/1 -> Add/1, M1/1
  Constant1/1 -> Add/2
  Add/1 -> M2/1

== system Modelo_Fuzzy_Manual/Main/A310 Model/WIND/Fuzzy alpha/Membership Function M ==
  vaz/vax1 : Inport
  Add3 : Sum
  Add4 : Sum
  Constant3 : Constant
  If : If  IfExpression=u1==0
  If Action Subsystem : Subsystem  TreatAsAtomicUnit=on
  If Action Subsystem1 : Subsystem  TreatAsAtomicUnit=on
  M1 : Outport
  M2 : Outport  Port=2
  wires:
  If/1 -> If Action Subsystem1/Action
  If/2 -> If Action Subsystem/Action
  Constant3/1 -> If Action Subsystem1/1(In1)
  If Action Subsystem1/1(M1) -> Add3/1
  If Action Subsystem1/2(M2) -> Add4/1
  Add3/1 -> M1/1
  Add4/1 -> M2/1
  If Action Subsystem/2(M2) -> Add4/2
  If Action Subsystem/1(M1) -> Add3/2
  vaz/vax1/1 -> If Action Subsystem/1(vaz/vax), If/1

== system Modelo_Fuzzy_Manual/Main/A310 Model/WIND/Fuzzy alpha/Membership Function N ==
  Vaz : Inport
  Vax : Inport  Port=2
  Add : Sum
  Add1 : Sum  Inputs=-+
  Constant : Constant  Value=400
  Constant1 : Constant  Value=800
  Constant2 : Constant
  Divide : Product  Inputs=*/
  Divide1 : Product  Inputs=*/
  N1 : Outport
  N2 : Outport  Port=2
  vaz/vax : Outport  Port=3
  wires:
  Vax/1 -> Divide/2
  Vaz/1 -> Divide/1
  Divide/1 -> vaz/vax/1, Add/2
  Constant/1 -> Add/1
  Add/1 -> Divide1/1
  Constant1/1 -> Divide1/2
  Divide1/1 -> Add1/1, N1/1
  Add1/1 -> N2/1
  Constant2/1 -> Add1/2

== system Modelo_Fuzzy_Manual/Main/A310 Model/Forces and Momments/Forces/CXYZ/Fuzzy CD (manual) ==
  alpha : Inport
  Add : Sum
  Add1 : Sum
  CD0 : Constant  Value=ACSP.COEF.CD.CD0
  CD_alpha : Gain  Gain=ACSP.COEF.CD.CDa
  CD_alpha1 : Gain  Gain=ParamFuzzy.CD.max
  CD_alpha2 : Gain  Gain=ACSP.COEF.CD.CDa2
  CD_alpha3 : Gain  Gain=ParamFuzzy.CD.min
  CD_alpha4 : Gain  Gain=ACSP.COEF.CD.CDa2
  Product : Product
  Product1 : Product
  Product2 : Product  Inputs=*/
  Sum2 : Sum  Inputs=+++
  mambership functions : Subsystem
  CD : Outport
  wires:
  CD_alpha2/1 -> CD_alpha1/1
  CD_alpha4/1 -> CD_alpha3/1
  alpha/1 -> CD_alpha/1, CD_alpha4/1, CD_alpha2/1, mambership functions/1(alpha)
  mambership functions/1(M1) -> Add1/1, Product/2
  CD_alpha1/1 -> Product/1
  mambership functions/2(M2) -> Add1/2, Product1/1
  CD_alpha3/1 -> Product1/2
  Product1/1 -> Add/2
  Product/1 -> Add/1
  Add/1 -> Product2/1
  Add1/1 -> Product2/2
  CD_alpha/1 -> Sum2/2
  CD0/1 -> Sum2/3
  Product2/1 -> Sum2/1
  Sum2/1 -> CD/1

== system Modelo_Fuzzy_Manual/Main/A310 Model/Forces and Momments/Forces/CXYZ/Fuzzy CL1 (manual) ==
  q : Inport
  Va : Inport  Port=2
  Add : Sum
  Add1 : Sum
  CLa4 : Gain  Gain=ACSP.COEF.CL.CLq
  CLa5 : Gain  Gain=ACSP.MIG.Lref
  Constant : Constant  Value=ParamFuzzy.CL1.min
  Constant1 : Constant  Value=ParamFuzzy.CL1.max
  Membership function M : Subsystem
  Product : Product  Inputs=*/
  Product1 : Product  Inputs=**
  Product2 : Product  Inputs=**
  Product3 : Product  Inputs=*/
  CL1 : Outport
  wires:
  q/1 -> Product/1
  Va/1 -> Product/2
  Product/1 -> Membership function M/1(q/Va)
  Membership function M/1(M1) -> Add1/1, Product1/2
  Membership function M/2(M2) -> Add1/2, Product2/1
  Constant/1 -> Product2/2
  Constant1/1 -> Product1/1
  Product2/1 -> Add/2
  Product1/1 -> Add/1
  Add/1 -> Product3/1
  Add1/1 -> Product3/2
  CLa4/1 -> CL1/1
  CLa5/1 -> CLa4/1
  Product3/1 -> CLa5/1

== system Modelo_Fuzzy_Manual/Main/A310 Model/Forces and Momments/Forces/CXYZ/Fuzzy CL2 (manual) ==
  Hlg : Inport
  Constant9 : Constant  Value=0
  If : If  IfExpression=u1 > 40
  If Action Subsystem : Subsystem  TreatAsAtomicUnit=on
  If Action Subsystem1 : Subsystem  TreatAsAtomicUnit=on
  Sum2 : Sum  Inputs=|++
  CL2 : Outport
  wires:
  If/2 -> If Action Subsystem1/Action
  If/1 -> If Action Subsystem/Action
  Constant9/1 -> If Action Subsystem/1(In1)
  If Action Subsystem/1(Out1) -> Sum2/1
  Sum2/1 -> CL2/1
  If Action Subsystem1/1(CL2) -> Sum2/2
  Hlg/1 -> If Action Subsystem1/1(Hlg), If/1

== system Modelo_Fuzzy_Manual/Main/A310 Model/Forces and Momments/Moments/Clmn/Cl ==
  U : Inport
  Bus Selector : BusSelector  OutputSignals=beta,p,Va,alpha,r,da,dr
  CD_alpha : Gain  Gain=ACSP.COEF.Cl.Clb
  CD_alpha3 : Gain  Gain=ACSP.COEF.Cl.Clda
  CD_alpha4 : Gain  Gain=ACSP.COEF.Cl.Cldr
  Fuzzy Cl1 (manual) : Subsystem
  Fuzzy Cl2 (manual) : Subsystem
  Sum1 : Sum
  Sum2 : Sum  Inputs=+++
  Sum3 : Sum
  Cl : Outport
  wires:
  Sum1/1 -> Sum2/3
  Sum2/1 -> Cl/1
  CD_alpha4/1 -> Sum1/2
  Bus Selector/1 -> CD_alpha/1  "<beta>"
  CD_alpha3/1 -> Sum1/1
  CD_alpha/1 -> Sum2/1
  Bus Selector/7 -> CD_alpha4/1  "<dr>"
  Bus Selector/6 -> CD_alpha3/1  "<da>"
  U/1 -> Bus Selector/1
  Sum3/1 -> Sum2/2
  Bus Selector/2 -> Fuzzy Cl1 (manual)/1(p)  "<p>"
  Bus Selector/5 -> Fuzzy Cl2 (manual)/3(r)  "<r>"
  Bus Selector/4 -> Fuzzy Cl2 (manual)/2(alpha)  "<alpha>"
  Bus Selector/3 -> Fuzzy Cl2 (manual)/1(Va), Fuzzy Cl1 (manual)/2(Va)  "<Va>"
  Fuzzy Cl1 (manual)/1(Cl1) -> Sum3/1
  Fuzzy Cl2 (manual)/1(Cl2) -> Sum3/2

== system Modelo_Fuzzy_Manual/Main/A310 Model/Forces and Momments/Moments/Clmn/Cm ==
  U : Inport
  Bus Selector : BusSelector  OutputSignals=alpha,q,Va,de
  Bus Selector3 : BusSelector  OutputSignals=Hlg,alpha
  CD_alpha : Gain  Gain=ACSP.COEF.Cm.Cma
  CD_alpha6 : Gain  Gain=ACSP.COEF.Cm.Cmde
  CL0 : Constant  Value=ACSP.COEF.Cm.Cm0
  Fuzzy Cm1 (manual) : Subsystem
  Fuzzy Cm2 (manual) : Subsystem
  Sum1 : Sum  Inputs=+++
  Sum2 : Sum  Inputs=|++
  Sum5 : Sum  Inputs=++|
  Cm : Outport
  wires:
  Sum2/1 -> Cm/1
  Sum5/1 -> Sum1/1
  CD_alpha6/1 -> Sum1/3
  CL0/1 -> Sum5/1
  CD_alpha/1 -> Sum5/2
  Sum1/1 -> Sum2/1
  Bus Selector/4 -> CD_alpha6/1  "<de>"
  Bus Selector/1 -> CD_alpha/1  "<alpha>"
  U/1 -> Bus Selector/1, Bus Selector3/1
  Fuzzy Cm1 (manual)/1(Cm1) -> Sum1/2
  Bus Selector/2 -> Fuzzy Cm1 (manual)/1(q)  "<q>"
  Bus Selector/3 -> Fuzzy Cm1 (manual)/2(Va)  "<Va>"
  Bus Selector3/2 -> Fuzzy Cm2 (manual)/2(alpha)  "<alpha>"
  Bus Selector3/1 -> Fuzzy Cm2 (manual)/1(Hlg)  "<Hlg>"
  Fuzzy Cm2 (manual)/1(Cm2) -> Sum2/2

== system Modelo_Fuzzy_Manual/Main/A310 Model/Forces and Momments/Moments/Clmn/Cn ==
  U : Inport
  Bus Selector : BusSelector  OutputSignals=beta,alpha,p,Va,r,da,dr
  CD_alpha3 : Gain  Gain=ACSP.COEF.Cn.Cnda
  CD_alpha4 : Gain  Gain=ACSP.COEF.Cn.Cndr
  Fuzzy Cn1 (manual) : Subsystem
  Fuzzy Cn2 (manual) : Subsystem
  Fuzzy Cn3 (manual) : Subsystem
  Sum1 : Sum
  Sum2 : Sum  Inputs=+++
  Sum3 : Sum
  Cn : Outport
  wires:
  Sum1/1 -> Sum2/3
  CD_alpha4/1 -> Sum1/2
  CD_alpha3/1 -> Sum1/1
  Bus Selector/7 -> CD_alpha4/1  "<dr>"
  Bus Selector/6 -> CD_alpha3/1  "<da>"
  Sum2/1 -> Cn/1
  U/1 -> Bus Selector/1
  Sum3/1 -> Sum2/2
  Bus Selector/2 -> Fuzzy Cn2 (manual)/1(alpha), Fuzzy Cn3 (manual)/2(alpha)  "<alpha>"
  Bus Selector/1 -> Fuzzy Cn3 (manual)/1(beta)  "<beta>"
  Fuzzy Cn1 (manual)/1(Cn1) -> Sum3/2
  Bus Selector/5 -> Fuzzy Cn1 (manual)/2(r)  "<r>"
  Bus Selector/4 -> Fuzzy Cn2 (manual)/3(Va), Fuzzy Cn1 (manual)/1(Va)  "<Va>"
  Fuzzy Cn2 (manual)/1(Cn2) -> Sum3/1
  Fuzzy Cn3 (manual)/1(Cn3) -> Sum2/1
  Bus Selector/3 -> Fuzzy Cn2 (manual)/2(p)  "<p>"

== system Modelo_Fuzzy_Manual/Main/A310 Model/WIND/Fuzzy Beta/Membership Function M/If Action Subsystem ==
  vay/va : Inport
  Action Port : ActionPort  ActionType=else
  Add : Sum  Inputs=-+
  Add1 : Sum  Inputs=-+
  Add2 : Sum  Inputs=-+
  Constant : Constant
  Constant1 : Constant  Value=pi/2
  Constant2 : Constant
  Divide : Product  Inputs=*/
  Divide1 : Product  Inputs=**
  Divide2 : Product  Inputs=**
  Trigonometric Function : Trigonometry  Operator=asin
  M1 : Outport
  M2 : Outport  Port=2
  wires:
  vay/va/1 -> Divide2/1, Add1/1, Divide1/2, Trigonometric Function/1
  Trigonometric Function/1 -> Add/2
  Constant/1 -> Divide1/1
  Divide1/1 -> Add/1
  Constant1/1 -> Divide2/2
  Divide2/1 -> Add1/2
  Add1/1 -> Divide/2
  Add/1 -> Divide/1
  Divide/1 -> Add2/1, M1/1
  Constant2/1 -> Add2/2
  Add2/1 -> M2/1

== system Modelo_Fuzzy_Manual/Main/A310 Model/WIND/Fuzzy Beta/Membership Function M/If Action Subsystem1 ==
  In1 : Inport
  Action Port : ActionPort  ActionType=then
  Constant : Constant  Value=0
  M1 : Outport
  M2 : Outport  Port=2
  wires:
  In1/1 -> M2/1
  Constant/1 -> M1/1

== system Modelo_Fuzzy_Manual/Main/A310 Model/WIND/Fuzzy alpha/Membership Function M/If Action Subsystem ==
  vaz/vax : Inport
  Action Port : ActionPort  ActionType=else
  Add : Sum  Inputs=-+
  Add1 : Sum  Inputs=+-
  Add2 : Sum  Inputs=-+
  Constant : Constant  Value=pi/800
  Constant1 : Constant  Value=pi/800
  Constant2 : Constant
  Divide : Product  Inputs=*/
  Divide1 : Product  Inputs=**
  Divide2 : Product  Inputs=**
  Trigonometric Function : Trigonometry  Operator=atan
  M1 : Outport
  M2 : Outport  Port=2
  wires:
  vaz/vax/1 -> Divide2/1, Add1/1, Divide1/2, Trigonometric Function/1
  Trigonometric Function/1 -> Add/2
  Constant/1 -> Divide1/1
  Divide1/1 -> Add/1
  Constant1/1 -> Divide2/2
  Divide2/1 -> Add1/2
  Add1/1 -> Divide/2
  Add/1 -> Divide/1
  Divide/1 -> Add2/1, M1/1
  Constant2/1 -> Add2/2
  Add2/1 -> M2/1

== system Modelo_Fuzzy_Manual/Main/A310 Model/WIND/Fuzzy alpha/Membership Function M/If Action Subsystem1 ==
  In1 : Inport
  Action Port : ActionPort  ActionType=then
  Constant : Constant  Value=0
  M1 : Outport
  M2 : Outport  Port=2
  wires:
  In1/1 -> M1/1
  Constant/1 -> M2/1

== system Modelo_Fuzzy_Manual/Main/A310 Model/Forces and Momments/Forces/CXYZ/Fuzzy CD (manual)/mambership functions ==
  alpha : Inport
  Constant : Constant  Value=ParamFuzzy.CD.max
  Constant1 : Constant
  Gain : Gain  Gain=1/(2*ParamFuzzy.CD.max)
  Sum : Sum  Inputs=|++
  Sum1 : Sum  Inputs=|-+
  M1 : Outport
  M2 : Outport  Port=2
  wires:
  alpha/1 -> Sum/1
  Constant/1 -> Sum/2
  Sum/1 -> Gain/1
  Gain/1 -> Sum1/1, M1/1
  Constant1/1 -> Sum1/2
  Sum1/1 -> M2/1

== system Modelo_Fuzzy_Manual/Main/A310 Model/Forces and Momments/Forces/CXYZ/Fuzzy CL1 (manual)/Membership function M ==
  q/Va : Inport
  Constant : Constant  Value=ParamFuzzy.CL1.min
  Constant1 : Constant  Value=ParamFuzzy.CL1.max
  Constant2 : Constant
  Product : Product  Inputs=*/
  Sum : Sum  Inputs=|+-
  Sum1 : Sum  Inputs=|-+
  Sum2 : Sum  Inputs=-+
  M1 : Outport
  M2 : Outport  Port=2
  wires:
  q/Va/1 -> Sum/1
  Constant/1 -> Sum1/1, Sum/2
  Sum/1 -> Product/1
  Sum1/1 -> Product/2
  Constant1/1 -> Sum1/2
  Product/1 -> Sum2/1, M1/1
  Constant2/1 -> Sum2/2
  Sum2/1 -> M2/1

== system Modelo_Fuzzy_Manual/Main/A310 Model/Forces and Momments/Forces/CXYZ/Fuzzy CL2 (manual)/If Action Subsystem ==
  In1 : Inport
  Action Port : ActionPort  InitializeStates=reset  ActionType=then
  Out1 : Outport
  wires:
  In1/1 -> Out1/1

== system Modelo_Fuzzy_Manual/Main/A310 Model/Forces and Momments/Forces/CXYZ/Fuzzy CL2 (manual)/If Action Subsystem1 ==
  Hlg : Inport
  Action Port : ActionPort  InitializeStates=reset  ActionType=else
  Add : Sum
  Add1 : Sum
  CLa1 : Gain  Gain=ACSP.COEF.CL.lambdah
  CLa2 : Gain  Gain=ACSP.COEF.CL.CLh
  Constant : Constant
  Constant1 : Constant
  Gain : Gain  Gain=-1/(2*ParamFuzzy.CL2.max)
  Product : Product
  Product1 : Product
  Product2 : Product  Inputs=*/
  Sum : Sum  Inputs=++|
  Sum1 : Sum  Inputs=|-+
  membership function M : Subsystem
  CL2 : Outport
  wires:
  Hlg/1 -> CLa1/1, Gain/1, membership function M/1(Hlg)
  membership function M/1(M1) -> Add1/1, Product/2
  membership function M/2(M2) -> Add1/2, Product1/1
  Gain/1 -> Sum/2
  Constant/1 -> Sum/1
  Sum/1 -> Product/1
  Constant1/1 -> Sum1/2
  Sum1/1 -> Product1/2
  Product/1 -> Add/1
  Product1/1 -> Add/2
  Add/1 -> Product2/1
  Add1/1 -> Product2/2
  Product2/1 -> CLa2/1
  CLa2/1 -> CL2/1
  CLa1/1 -> Sum1/1

== system Modelo_Fuzzy_Manual/Main/A310 Model/Forces and Momments/Moments/Clmn/Cl/Fuzzy Cl1 (manual) ==
  p : Inport
  Va : Inport  Port=2
  Add : Sum
  Add1 : Sum
  CLa4 : Gain  Gain=ACSP.COEF.Cl.Clp
  CLa5 : Gain  Gain=ACSP.MIG.Lref
  Constant : Constant  Value=ParamFuzzy.Cl1.min
  Constant1 : Constant  Value=ParamFuzzy.Cl1.max
  Membership function M : Subsystem
  Product : Product  Inputs=*/
  Product1 : Product  Inputs=**
  Product2 : Product  Inputs=**
  Product3 : Product  Inputs=*/
  Cl1 : Outport
  wires:
  p/1 -> Product/1
  Va/1 -> Product/2
  Product/1 -> Membership function M/1(p/Va)
  Membership function M/1(M1) -> Add1/1, Product1/2
  Membership function M/2(M2) -> Add1/2, Product2/1
  Constant/1 -> Product2/2
  Constant1/1 -> Product1/1
  Product2/1 -> Add/2
  Product1/1 -> Add/1
  Add/1 -> Product3/1
  Add1/1 -> Product3/2
  CLa5/1 -> CLa4/1
  Product3/1 -> CLa5/1
  CLa4/1 -> Cl1/1

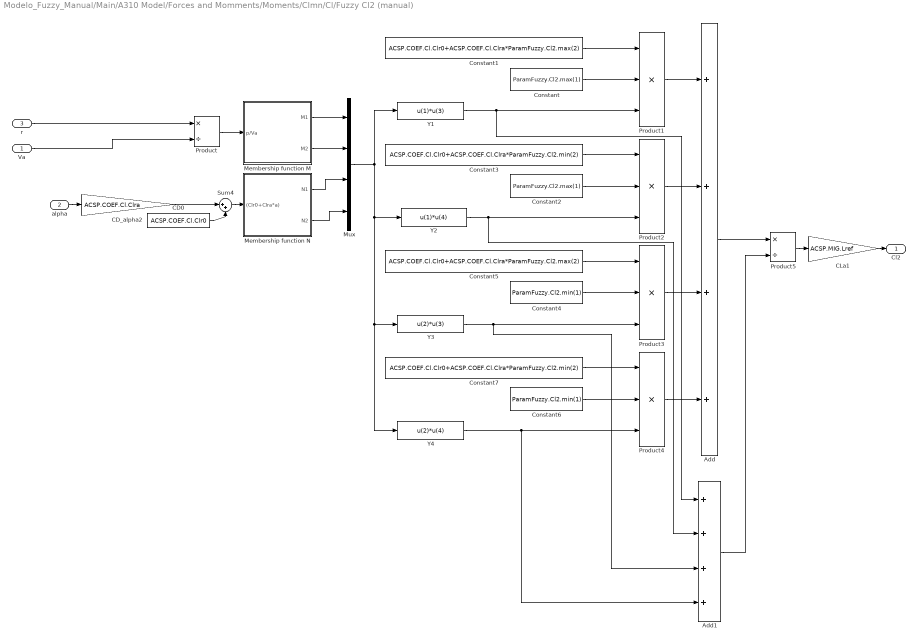
== system Modelo_Fuzzy_Manual/Main/A310 Model/Forces and Momments/Moments/Clmn/Cl/Fuzzy Cl2 (manual) ==
  Va : Inport
  alpha : Inport  Port=2
  r : Inport  Port=3
  Add : Sum  Inputs=++++
  Add1 : Sum  Inputs=++++
  CD0 : Constant  Value=ACSP.COEF.Cl.Clr0
  CD_alpha2 : Gain  Gain=ACSP.COEF.Cl.Clra
  CLa1 : Gain  Gain=ACSP.MIG.Lref
  Constant : Constant  Value=ParamFuzzy.Cl2.max(1)
  Constant1 : Constant  Value=ACSP.COEF.Cl.Clr0+ACSP.COEF.Cl.Clra*ParamFuzzy.Cl2.max(2)
  Constant2 : Constant  Value=ParamFuzzy.Cl2.max(1)
  Constant3 : Constant  Value=ACSP.COEF.Cl.Clr0+ACSP.COEF.Cl.Clra*ParamFuzzy.Cl2.min(2)
  Constant4 : Constant  Value=ParamFuzzy.Cl2.min(1)
  Constant5 : Constant  Value=ACSP.COEF.Cl.Clr0+ACSP.COEF.Cl.Clra*ParamFuzzy.Cl2.max(2)
  Constant6 : Constant  Value=ParamFuzzy.Cl2.min(1)
  Constant7 : Constant  Value=ACSP.COEF.Cl.Clr0+ACSP.COEF.Cl.Clra*ParamFuzzy.Cl2.min(2)
  Membership function M : Subsystem
  Membership function N : Subsystem
  Mux : Mux
  Product : Product  Inputs=*/
  Product{1..4} (4 alike) : Product  Inputs=***
  Product5 : Product  Inputs=*/
  Sum4 : Sum  Inputs=|++
  Y1 : Fcn  Expr=u(1)*u(3)
  Y2 : Fcn  Expr=u(1)*u(4)
  Y3 : Fcn  Expr=u(2)*u(3)
  Y4 : Fcn  Expr=u(2)*u(4)
  Cl2 : Outport
  wires:
  r/1 -> Product/1
  Va/1 -> Product/2
  Product/1 -> Membership function M/1(p/Va)
  CD0/1 -> Sum4/2
  CD_alpha2/1 -> Sum4/1
  alpha/1 -> CD_alpha2/1
  Sum4/1 -> Membership function N/1((Clr0+Clra*a))
  Membership function M/1(M1) -> Mux/1
  Membership function M/2(M2) -> Mux/2
  Membership function N/1(N1) -> Mux/3
  Membership function N/2(N2) -> Mux/4
  Mux/1 -> Y4/1, Y3/1, Y2/1, Y1/1
  Constant1/1 -> Product1/1
  Constant/1 -> Product1/2
  Y1/1 -> Add1/1, Product1/3
  Constant3/1 -> Product2/1
  Constant2/1 -> Product2/2
  Y2/1 -> Add1/2, Product2/3
  Constant5/1 -> Product3/1
  Constant4/1 -> Product3/2
  Y3/1 -> Add1/3, Product3/3
  Constant7/1 -> Product4/1
  Constant6/1 -> Product4/2
  Y4/1 -> Add1/4, Product4/3
  Product4/1 -> Add/4
  Product3/1 -> Add/3
  Product1/1 -> Add/1
  Product2/1 -> Add/2
  Add/1 -> Product5/1
  Add1/1 -> Product5/2
  Product5/1 -> CLa1/1
  CLa1/1 -> Cl2/1
